simulink model "projekat_model"  (R2025a)
settings: Solver=VariableStepAuto  StartTime=0.0  StopTime=5000  RelTol=1e-3
undefined symbols (not defined in the file): Tf
settings Model: Creator=neso  LastModifiedBy=Korisnik

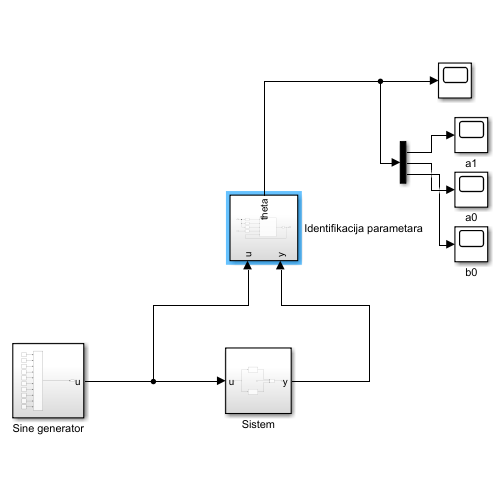
[thumbnail: Simulink's stored preview of the top-level diagram]
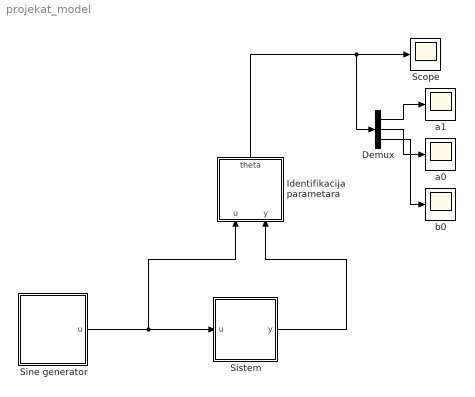
== system projekat_model ==
  Demux : Demux  Outputs=3
  Identifikacija parametara : Subsystem
  Scope : Scope
      settings: ActiveDisplayYMinimum=-14.891910412478707  ActiveDisplayYMaximum=20.065851973385055
  Sine generator : Subsystem
  Sistem : Subsystem
  a0 : Scope
      settings: ActiveDisplayYMinimum=-8.5109294559908086  ActiveDisplayYMaximum=21.084373521888086  DataLoggingVariableName=ScopeData2
  a1 : Scope
      settings: ActiveDisplayYMinimum=0.935675841003011  ActiveDisplayYMaximum=9.3006227399808985
  b0 : Scope
      settings: ActiveDisplayYMinimum=-8.5109294559908086  ActiveDisplayYMaximum=21.084373521888086  DataLoggingVariableName=ScopeData3
  wires:
  Sistem/1(y) -> Identifikacija parametara/2(y)
  Identifikacija parametara/1(theta) -> Demux/1, Scope/1
  Sine generator/1(u) -> Identifikacija parametara/1(u), Sistem/1(u)
  Demux/1 -> a1/1
  Demux/2 -> a0/1
  Demux/3 -> b0/1

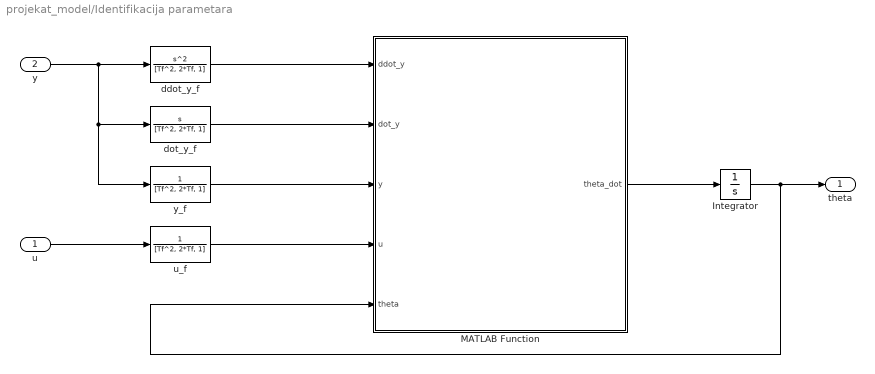
== system projekat_model/Identifikacija parametara ==
  u : Inport
  y : Inport  Port=2
  Integrator : Integrator  InitialCondition=[0; 0; 0]
  MATLAB Function : MATLAB Function  TreatAsAtomicUnit=on
  ddot_y_f : TransferFcn  Numerator=[1, 0, 0]  Denominator=[Tf^2, 2*Tf, 1]
  dot_y_f : TransferFcn  Numerator=[1, 0]  Denominator=[Tf^2, 2*Tf, 1]
  u_f : TransferFcn  Denominator=[Tf^2, 2*Tf, 1]
  y_f : TransferFcn  Denominator=[Tf^2, 2*Tf, 1]
  theta : Outport
  wires:
  y/1 -> y_f/1, dot_y_f/1, ddot_y_f/1
  u/1 -> u_f/1
  ddot_y_f/1 -> MATLAB Function/1(ddot_y)
  dot_y_f/1 -> MATLAB Function/2(dot_y)
  y_f/1 -> MATLAB Function/3(y)
  u_f/1 -> MATLAB Function/4(u)
  MATLAB Function/1(theta_dot) -> Integrator/1
  Integrator/1 -> MATLAB Function/5(theta), theta/1

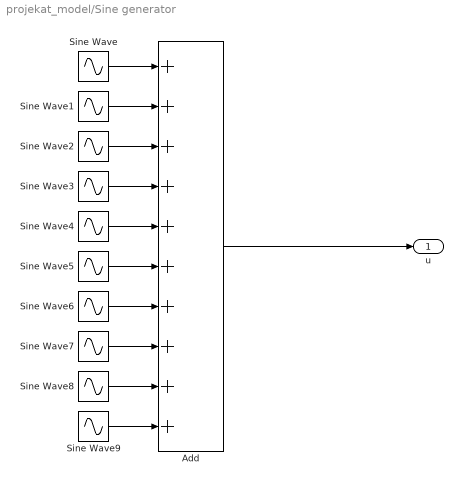
== system projekat_model/Sine generator ==
  Add : Sum  Inputs=10
  Sine Wave : Sin  SampleTime=0
  Sine Wave1 : Sin  Frequency=2  SampleTime=0
  Sine Wave2 : Sin  Frequency=3  SampleTime=0
  Sine Wave3 : Sin  Frequency=4  SampleTime=0
  Sine Wave4 : Sin  Frequency=5  SampleTime=0
  Sine Wave5 : Sin  Frequency=6  SampleTime=0
  Sine Wave6 : Sin  Frequency=7  SampleTime=0
  Sine Wave7 : Sin  Frequency=8  SampleTime=0
  Sine Wave8 : Sin  Frequency=9  SampleTime=0
  Sine Wave9 : Sin  Frequency=10  SampleTime=0
  u : Outport
  wires:
  Add/1 -> u/1
  Sine Wave/1 -> Add/1
  Sine Wave1/1 -> Add/2
  Sine Wave2/1 -> Add/3
  Sine Wave3/1 -> Add/4
  Sine Wave4/1 -> Add/5
  Sine Wave5/1 -> Add/6
  Sine Wave6/1 -> Add/7
  Sine Wave7/1 -> Add/8
  Sine Wave8/1 -> Add/9
  Sine Wave9/1 -> Add/10

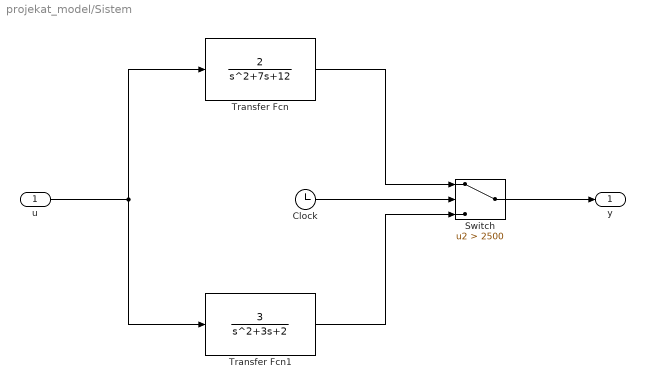
== system projekat_model/Sistem ==
  u : Inport
  Clock : Clock
  Switch : Switch  Criteria=u2 > Threshold  Threshold=2500  SaturateOnIntegerOverflow=off  InputSameDT=off
  Transfer Fcn : TransferFcn  Numerator=[2]  Denominator=[1, 7, 12]
  Transfer Fcn1 : TransferFcn  Numerator=3  Denominator=[1, 3, 2]
  y : Outport
  wires:
  u/1 -> Transfer Fcn1/1, Transfer Fcn/1
  Transfer Fcn/1 -> Switch/1
  Transfer Fcn1/1 -> Switch/3
  Switch/1 -> y/1
  Clock/1 -> Switch/2

== matlab function projekat_model/Identifikacija parametara/MATLAB Function ==
  data: ddot_y input; dot_y input; y input; u input; theta_dot output; theta input
function theta_dot = fcn(ddot_y, dot_y, y, u, theta)
    p = [-dot_y; -y; u];
    eta = ddot_y;
    
    G = 0.2 * eye(length(p), length(p));
    theta_dot = G * p * (eta - p' * theta);
end
